simulink model "PMMUnderActuated_1stgen_invPend"  (R2013a)
settings: Solver=ode45  StartTime=0.0  StopTime=t_final  MaxStep=1e-2  RelTol=1e-3
values from neighbouring files (symbols this model uses):
  g = 9.81    [PMMUnderActuated_1stgen_init.m]
  I_t = 1.4    [PMMUnderActuated_1stgen_init.m]
  xt_des = 0    [PMMUnderActuated_1stgen_init.m]
undefined symbols (not defined in the file or in its folder): kdx, kpx, l_pend, m_pend
libraries: mblibv1 x8
settings Model: Creator=hgeyer  LastModifiedBy=benshih
settings SolverCC: ZeroCrossAlgorithm=Adaptive
settings DataIOCC: LimitDataPoints=off  SignalLoggingSaveFormat=ModelDataLogs
settings OptimizationCC: ExpressionDepthLimit=2147483647
settings DebuggingCC: FcnCallInpInsideContextMsg=EnableAllAsWarning
settings GRTTargetCC: CombineOutputUpdateFcns=off  GRTInterface=on
settings SimMechanicsCC: VisOnUpdateDiagram=on  VisDuringSimulation=on  VisSampleTime=0.01  LastVizWinPosition=[360 260 560 420]  CamPosition=[-0.0148721;0.526751;11.5664;]  CamTarget=[-0.124996;0.5;-2.10125e-06;]  CamUpVector=[0.00454429;0.999987;-0.00235607;]  CamHeight=1.02  VisBackgroundColor=[0.9;0.9;0.95;]  DefaultBodyColor=[1;0;0;]

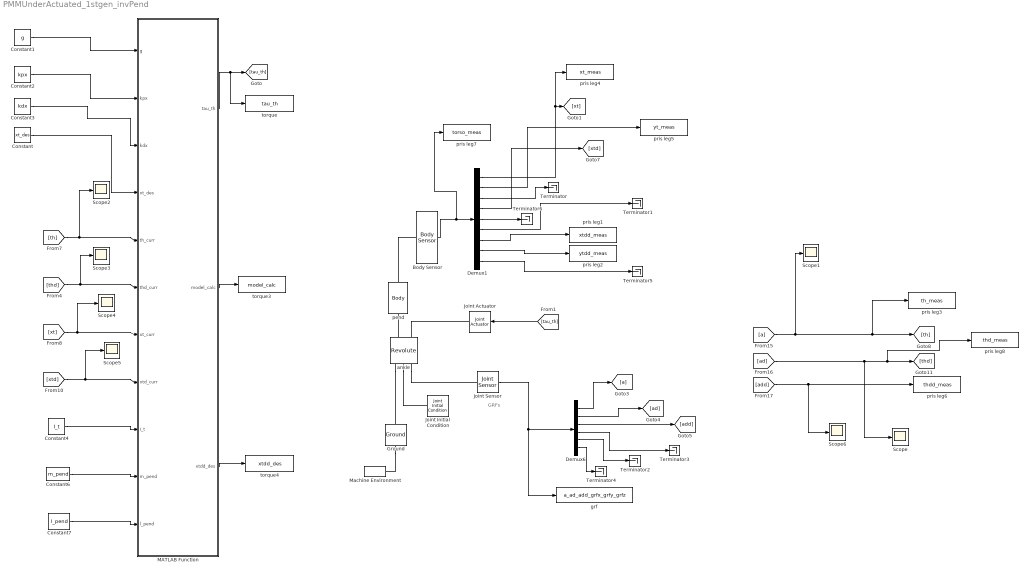
== system PMMUnderActuated_1stgen_invPend ==
  note: GRFs
  Body Sensor : mblibv1/Sensors &  Actuators/Body Sensor  UpdateFromCAD=off  PhysicalDomain=Mechanical  PortType=blob  Muxed=on  Pose=off  Angle=on  AngleUnits=deg  ArcVelocity=off  ArcVelocityUnits=deg/s  ArcAcceleration=off  ArcAccelerationUnits=deg/s^2  CoordPosition=on  CoordPositionUnits=m  Velocity=on  VelocityUnits=m/s  Acceleration=on  AccelerationUnits=m/s^2  Quaternion=on  QuaternionDT=off  QuaternionDDT=off  QuaternionUnits=off  OutputVector=[1]  ActiveIO=on  Width=9  DialogClass=MechanicalSensorBlock  ReferenceFrame=Absolute (World)
  Constant : Constant  Value=xt_des
  Constant1 : Constant  Value=g
  Constant2 : Constant  Value=kpx
  Constant3 : Constant  Value=kdx
  Constant4 : Constant  Value=I_t
  Constant6 : Constant  Value=m_pend
  Constant7 : Constant  Value=l_pend
  Demux1 : Demux  Outputs=9
  Demux6 : Demux  Outputs=6
  Ground : mblibv1/Bodies/Ground  UpdateFromCAD=off  LeftPortType=env  RightPortType=workingframe  PhysicalDomain=Mechanical  DialogClass=GroundBlock  CoordPosition=[0 0 0]  CoordPositionUnits=m  StateVectorMgrId=0  MachineId=[1 0]  ShowEnvPort=on
  Joint Actuator : mblibv1/Sensors &  Actuators/Joint Actuator  UpdateFromCAD=off  PhysicalDomain=Mechanical  PortType=blob  ActuationStyle=Force  AngleUnits=deg  ArcVelocityUnits=deg/s  ArcAccelerationUnits=deg/s^2  CoordPositionUnits=m  VelocityUnits=m/s  AccelerationUnits=m/s^2  ForceUnits=N  TorqueUnits=N*m  ActiveIO=on  Width=1  DialogClass=MechanicalActuatorBlock  Primitive=R1  ReferenceFrame=Absolute (World)
  Joint Initial Condition : mblibv1/Sensors &  Actuators/Joint Initial Condition  UpdateFromCAD=off  LeftPortType=blob  RightPortType=blob  PhysicalDomain=mechanical  DialogClass=InitialConditionBlock  InitialConditions=P1$false$0$m$deg$0$m/s$deg/s#P2$false$0$m$deg$0$m/s$deg/s#P3$false$0$m$deg$0$m/s$deg/s#R1$true$th_angle_init$m$rad$0$m/s$rad/s#R2$false$0$m$deg$0$m/s$deg/s#R3$false$0$m$deg$0$m/s$deg/s#S$false$0$m$deg$0$m/s$deg/s  P1PIC=0  P1VIC=0  P2PIC=0  P2VIC=0  P3PIC=0  P3VIC=0  R1PIC=th_angle_init  R1VIC=0  R2PIC=0  R2VIC=0  R3PIC=0  R3VIC=0  SPIC=0  SVIC=0
  Joint Sensor : mblibv1/Sensors &  Actuators/Joint Sensor  UpdateFromCAD=off  PhysicalDomain=Mechanical  PortType=blob  Muxed=on  Pose=off  Angle=on  AngleUnits=rad  ArcVelocity=on  ArcVelocityUnits=rad/s  ArcAcceleration=on  ArcAccelerationUnits=rad/s^2  CoordPosition=on  CoordPositionUnits=m  Velocity=off  VelocityUnits=m/s  Acceleration=off  AccelerationUnits=m/s^2  Quaternion=on  QuaternionDT=off  QuaternionDDT=off  QuaternionUnits=off  OutputVector=[1]  ActiveIO=on  Width=6  DialogClass=MechanicalSensorBlock  Primitive=R1  Force=off  ForceUnits=N  Torque=off  TorqueUnits=N*m  ReferenceFrame=Absolute (World)  ReactionSensedSide=Follower  ReactionReferenceFrame=Absolute (World)  ReactionForce=on  ReactionForceUnits=N  ReactionMoment=off  ReactionMomentUnits=N*m
  MATLAB Function : MATLAB Function  TreatAsAtomicUnit=on
  Machine Environment : mblibv1/Bodies/Machine Environment  PortType=env  PhysicalDomain=Mechanical  DialogTemplateClass=MECH.MachineEnvironment  SyncWhenCopied=off  Gravity=[0 -9.81 0]  GravityUnits=m/s^2  GravityAsSignal=off  Dimensionality=2D Only  AnalysisType=Forward dynamics  LinearAssemblyTolerance=1e-3  LinearAssemblyToleranceUnits=m  AngularAssemblyTolerance=1e-3  AngularAssemblyToleranceUnits=rad  ConstraintSolverType=Stabilizing  ConstraintRelTolerance=1e-4  ConstraintAbsTolerance=1e-4  UseRobustSingularityHandling=off  RedundancyAnalysisToleranceType=Automatically select tolerance  RedundancyAnalysisTolerance=1e-14  StatePerturbationType=Fixed  PerturbationSize=1e-5  VisualizeMachine=on  BodyVisualizationType=Use model default body geometries  BodyColorSelMode=Use model default  DefaultBodyColor=[1 0 0]
  Scope{,1..6} (7 alike) : Scope
      Scope2 settings: SaveName=ScopeData2
      Scope3 settings: SaveName=ScopeData3
      Scope4 settings: SaveName=ScopeData4
      Scope5 settings: SaveName=ScopeData5
      Scope6 settings: SaveName=ScopeData6
  Terminator{,1..6} (7 alike) : Terminator
  ankle : mblibv1/Joints/Revolute  LConnTagsString=__newl0|SA1|SA2  RConnTagsString=__newr0|SA1  UpdateFromCAD=off  NumSAPorts=3  CutJoint=off  MarkAsCut=off  Primitives=prismatic  PrimitiveProps=R1$World$[0 0 -1]$revolute  DialogClass=JointBlock  R1Axis=[0 0 -1]
  grf : ToWorkspace  VariableName=a_ad_add_grfx_grfy_grfz  SampleTime=-1
  pend : mblibv1/Bodies/Body  LConnTagsString=CS1  RConnTagsString=CS2  UpdateFromCAD=off  DialogClass=MechanicalBodyBlock  Mass=m_pend  MassUnits=kg  InertiaUnits=kg*m^2  Inertia=[0 0 0; 0 0 0; 0 0 -I_t]  Shape=Cylinder  ShapeDims=[1 1]  ShapeUnits=m  ShapeUse=false  Density=1  DensityUnits=kg/m^3  DensityUse=false  GraphicsMode=MACHINE_DEFAULT  BodyColorSelMode=MACHINE_DEFAULT  BodyColor=[1 0 0]  AttachedToCS=CG  CG=Left$CG$[0 l_pend 0]$CS1$CS1$m$[0 0 0]$Euler X-Y-Z$deg$WORLD$false$none  WorkingFrames=Left$CS1$[0 0 0]$Adjoining$Adjoining$m$[0 0 0]$Euler X-Y-Z$deg$WORLD$true$none#Right$CS2$[0 l_pend 0]$CS1$CS1$m$[0 0 0]$Euler X-Y-Z$deg$WORLD$true$none  CGPos=[0 l_pend 0]  CGRot=[0 0 0]  CS0Pos=[]  CS0Rot=[]  CS1Pos=[0 0 0]  CS1Rot=[0 0 0]  CS2Pos=[0 l_pend 0]  CS2Rot=[0 0 0]  CS3Pos=[]  CS3Rot=[]  CS4Pos=[]  CS4Rot=[]  CS5Pos=[]  CS5Rot=[]  CS6Pos=[]  CS6Rot=[]  CS7Pos=[]  CS7Rot=[]  CS8Pos=[]  CS8Rot=[]  CS9Pos=[]  CS9Rot=[]  CS10Pos=[]  CS10Rot=[]  CS11Pos=[]  CS11Rot=[]  CS12Pos=[]  CS12Rot=[]  CS13Pos=[]  CS13Rot=[]  CS14Pos=[]  CS14Rot=[]  CS15Pos=[]  CS15Rot=[]  CS16Pos=[]  CS16Rot=[]  CS17Pos=[]  CS17Rot=[]  CS18Pos=[]  CS18Rot=[]  CS19Pos=[]  CS19Rot=[]  CS20Pos=[]  CS20Rot=[]
  pris leg1 : ToWorkspace  VariableName=xtdd_meas  SampleTime=-1
  pris leg2 : ToWorkspace  VariableName=ytdd_meas  SampleTime=-1
  pris leg3 : ToWorkspace  VariableName=th_meas  SampleTime=-1
  pris leg4 : ToWorkspace  VariableName=xt_meas  SampleTime=-1
  pris leg5 : ToWorkspace  VariableName=yt_meas  SampleTime=-1
  pris leg6 : ToWorkspace  VariableName=thdd_meas  SampleTime=-1
  pris leg7 : ToWorkspace  VariableName=torso_meas  SampleTime=-1
  pris leg8 : ToWorkspace  VariableName=thd_meas  SampleTime=-1
  torque : ToWorkspace  VariableName=tau_th  SampleTime=-1
  torque3 : ToWorkspace  VariableName=model_calc  SampleTime=-1
  torque4 : ToWorkspace  VariableName=xtdd_des  SampleTime=-1
  wires:
  MATLAB Function/1(tau_th) -> torque/1, [tau_th]
  Constant/1 -> MATLAB Function/4(xt_des)
  [xt] -> Scope4/1, MATLAB Function/7(xt_curr)
  [th] -> Scope2/1, MATLAB Function/5(th_curr)
  MATLAB Function/2(model_calc) -> torque3/1
  MATLAB Function/3(xtdd_des) -> torque4/1
  Joint Sensor/1 -> Demux6/1, grf/1
  Demux6/5 -> Terminator2/1
  Demux6/4 -> Terminator3/1
  Demux6/1 -> [a]
  Demux6/2 -> [ad]
  Demux6/6 -> Terminator4/1
  Demux6/3 -> [add]
  Constant4/1 -> MATLAB Function/9(I_t)
  Constant7/1 -> MATLAB Function/11(l_pend)
  Constant6/1 -> MATLAB Function/10(m_pend)
  Demux1/3 -> Terminator/1
  Demux1/9 -> Terminator5/1
  Demux1/6 -> Terminator1/1
  Demux1/4 -> [xtd]
  Demux1/1 -> pris leg4/1, [xt]
  Demux1/2 -> pris leg5/1
  Demux1/7 -> pris leg1/1
  Demux1/8 -> pris leg2/1
  Body Sensor/1 -> pris leg7/1, Demux1/1
  [a] -> Scope1/1, pris leg3/1, [th]
  [ad] -> Scope/1, pris leg8/1, [thd]
  [add] -> Scope6/1, pris leg6/1
  Constant1/1 -> MATLAB Function/1(g)
  Constant2/1 -> MATLAB Function/2(kpx)
  Constant3/1 -> MATLAB Function/3(kdx)
  Demux1/5 -> Terminator6/1
  [thd] -> Scope3/1, MATLAB Function/6(thd_curr)
  [xtd] -> Scope5/1, MATLAB Function/8(xtd_curr)
  [tau_th] -> Joint Actuator/1
  connections:
  Ground/LConn1 -- Machine Environment/RConn1
  ankle/LConn2 -- Joint Initial Condition/RConn1
  ankle/LConn3 -- Joint Sensor/LConn1
  ankle/LConn1 -- Ground/RConn1
  ankle/RConn1 -- pend/LConn1
  pend/RConn1 -- Body Sensor/LConn1
  ankle/RConn2 -- Joint Actuator/RConn1

== matlab function PMMUnderActuated_1stgen_invPend/MATLAB Function ==
  data: g input; kpx input; kdx input; tau_th output; model_calc output; xt_des input; th_curr input; thd_curr input; xt_curr input; xtd_curr input; xtdd_des output; I_t input; m_pend input; l_pend input
function [tau_th, model_calc, xtdd_des] = MotorTorqueEvaluation(g, kpx, kdx, xt_des, th_curr, thd_curr, xt_curr, xtd_curr, I_t, m_pend, l_pend)


    % Desired accelerations. xtd, ytd, thd are 0.
    xtdd_des = kpx*(xt_curr - xt_des) + kdx*(xtd_curr);
    
    % Rearranging the equations as Ax = b and solving. Assumes Tth = 0.
    A = [1 0 I_t -l_pend*cos(th_curr) l_pend*sin(th_curr);
         0 0 0 1 0;
         0 -m_pend 0 0 1;
         0 0 l_pend*cos(th_curr) 0 0;
         0 1 l_pend*sin(th_curr) 0 0];

     b = [0
          m_pend*xtdd_des;
          -m_pend*g;
          xtdd_des + l_pend * sin(th_curr)*thd_curr^2;
          -l_pend * cos(th_curr)*thd_curr^2];
     
    % Solve for the unknown values x = [T_th, ytdd, thdd, GRFx, GRFy]'
    x = A^-1*b;

    tau_th = x(1);
    model_calc = x;

end
